simulink model "PackMLStateFlow"  (R2022b)
settings: Solver=ode3  StartTime=0.0  StopTime=Inf  RelTol=1e-3
settings Model: Creator=ChrisK  LastModifiedBy=ChrisK
settings OptimizationCC: DefaultParameterBehavior=Inlined  LocalBlockOutputs=off
settings RTWCC: Description=TwinCAT GRT Target  SystemTargetFile=TwinCatGrt.tlc  GenCodeOnly=on  GenerateMakefile=off  TemplateMakefile=tcgrt_msbuild.tmf  TargetLang=C++
settings STFCustomTargetCC: TargetLangStandard=C++11 (ISO)  ConcurrentExecutionCompliant=on  CombineOutputUpdateFcns=on  CodeInterfacePackaging=Reusable function  CPPClassGenCompliant=on  GenerateAllocFcn=on  SystemTargetFile=TwinCatGrt.tlc
settings GRTTargetCC: TargetLangStandard=C++11 (ISO)  ParMdlRefBuildCompliant=off  CompOptLevelCompliant=off  MatFileLogging=off  CodeInterfacePackaging=Reusable function  GenerateAllocFcn=on  UseToolchainInfoCompliant=off  ExtModeMexFile=TcExtModeClient

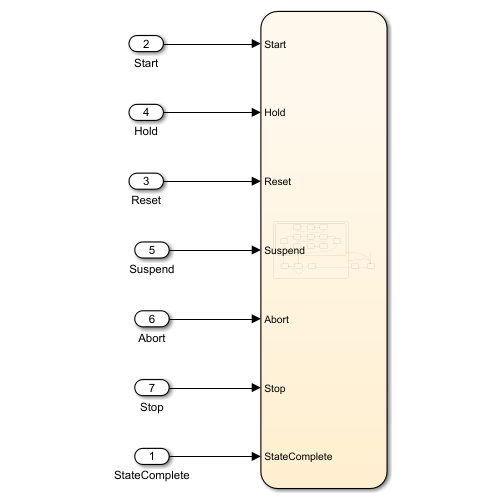
[thumbnail: Simulink's stored preview of the top-level diagram]
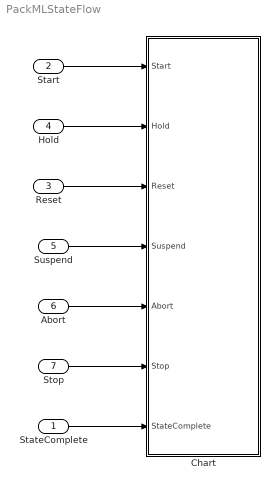
== system PackMLStateFlow ==
  StateComplete : Inport  OutDataTypeStr=boolean
  Start : Inport  Port=2  OutDataTypeStr=boolean
  Reset : Inport  Port=3  OutDataTypeStr=boolean
  Hold : Inport  Port=4  OutDataTypeStr=boolean
  Suspend : Inport  Port=5  OutDataTypeStr=boolean
  Abort : Inport  Port=6  OutDataTypeStr=boolean
  Stop : Inport  Port=7  OutDataTypeStr=boolean
  Chart : Stateflow chart  TreatAsAtomicUnit=on
  wires:
  StateComplete/1 -> Chart/7(StateComplete)
  Start/1 -> Chart/1(Start)
  Reset/1 -> Chart/3(Reset)
  Hold/1 -> Chart/2(Hold)
  Suspend/1 -> Chart/4(Suspend)
  Abort/1 -> Chart/5(Abort)
  Stop/1 -> Chart/6(Stop)

== stateflow chart PackMLStateFlow/Chart ==
  state Abortable
    state Stoppable
      state UnHolding
      state Held
      state Holding
      state Starting
      state Execute
      state Completing
      state Idle
      state Complete
      state UnSuspending
      state Suspended
      state Suspending
      state Resetting
      Held -> UnHolding : [Start == true]
      Holding -> Held : [StateComplete == true]
      UnHolding -> Execute : [StateComplete == true]
      Execute -> Holding [order 2] : [Hold == true]
      Completing -> Complete : [StateComplete == true]
      Idle -> Starting : [Start == true]
      Starting -> Execute : [StateComplete == true]
      Execute -> Completing [order 1] : [Complete == true]
      UnSuspending -> Execute : [StateComplete == true]
      Execute -> Suspending [order 3] : [Suspend == true]
      Resetting -> Idle : [StateComplete == true]
      Complete -> Resetting : [Reset == true]
      Suspended -> UnSuspending : [Start == true]
      Suspending -> Suspended : [StateComplete == true]
    state Stopped
    state Stopping
    state Clearing
    Stopped -> Resetting : [Reset == true]
    Stoppable -> Stopping [order 1] : [Stop == true]
    Clearing -> Stopped : [StateComplete == true]
    Stopping -> Stopped : [StateComplete == true]
  state Aborted
  state Aborting
  (default) -> Aborting
  Stoppable -> Aborting [order 2] : [Abort == true]
  Abortable -> Aborting : [Abort == true]
  Aborted -> Clearing : [Reset == true]
  Aborting -> Aborted : [StateComplete == true]
  data: Start input; Hold input; Reset input; Suspend input; Abort input; Stop input; StateComplete input
